simulink model "QSS_Tutor"  (R2025a)
settings: Solver=VariableStepAuto  StartTime=0.0  StopTime=231  RelTol=1e-3
libraries: qss_tb_library x2
settings Model: Creator=venich  LastModifiedBy=venich

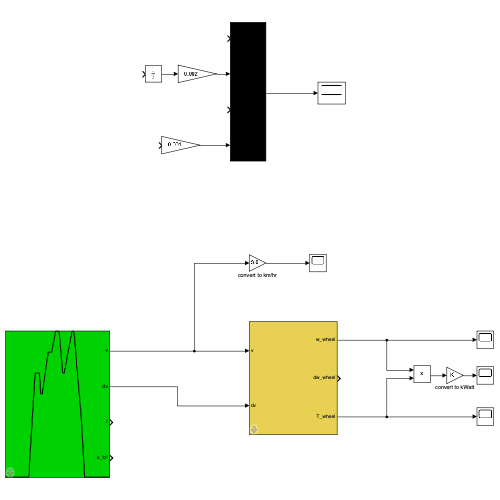
[thumbnail: Simulink's stored preview of the top-level diagram]
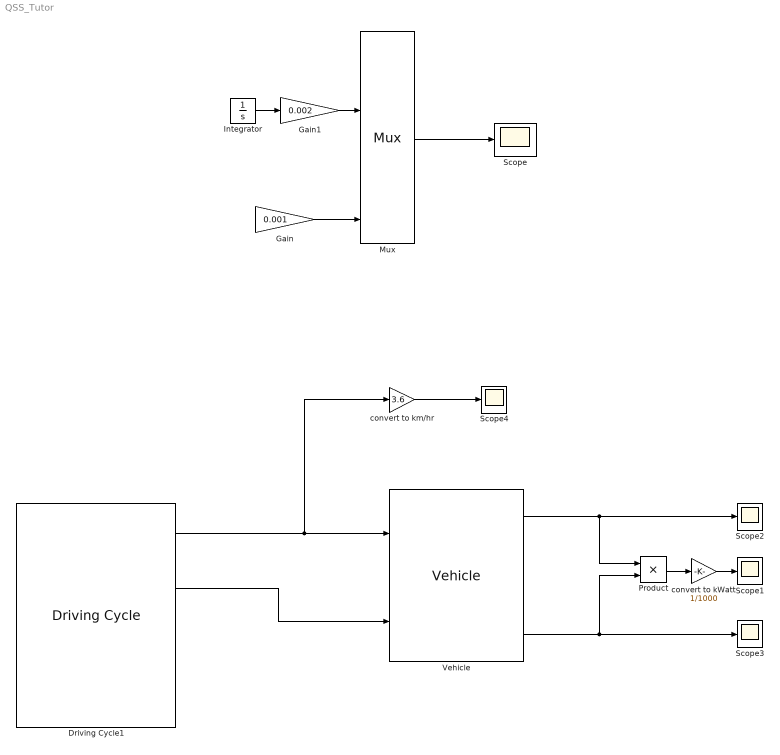
== system QSS_Tutor ==
  Driving Cycle1 : qss_tb_library/Driving Cycle/Driving Cycle  Tag=cycle  cyclenr="Japan:  15-Mode"  stepsize=1  autostop=on
  Gain : Gain  Gain=0.001
  Gain1 : Gain  Gain=0.002
  Integrator : Integrator
  Mux : Mux
  Product : Product
  Scope{,1..4} (5 alike) : Scope
      Scope settings: ActiveDisplayYMinimum=-4.1666666666666661  ActiveDisplayYMaximum=37.5
      Scope1 settings: ActiveDisplayYMinimum=-16.799987804789673  ActiveDisplayYMaximum=22.505354826441003
      Scope2 settings: ActiveDisplayYMinimum=-7978.7783692887479  ActiveDisplayYMaximum=11525.451449900802  DataLoggingVariableName=ScopeData2
      Scope3 settings: ActiveDisplayYMinimum=-7978.7783692887479  ActiveDisplayYMaximum=11525.451449900802  DataLoggingVariableName=ScopeData3
      Scope4 settings: ActiveDisplayYMinimum=-8.7499999999999982  ActiveDisplayYMaximum=78.75  DataLoggingVariableName=ScopeData4
  Vehicle : qss_tb_library/Vehicle/Vehicle  Tag=vehicle  m_f=1500  mt2m_f=5  A_f=1.8  d_wheel=0.5  cw=0.22  mu=0.008
  convert to kWatt : Gain  Gain=1/1000
  convert to km/hr : Gain  Gain=3.6
  wires:
  Mux/1 -> Scope/1
  Gain/1 -> Mux/4
  Integrator/1 -> Gain1/1
  Gain1/1 -> Mux/2
  Driving Cycle1/1 -> Vehicle/1, convert to km/hr/1
  Driving Cycle1/2 -> Vehicle/2
  Vehicle/1 -> Product/1, Scope2/1
  Vehicle/3 -> Product/2, Scope3/1
  Product/1 -> convert to kWatt/1
  convert to kWatt/1 -> Scope1/1
  convert to km/hr/1 -> Scope4/1
